simulink model "TestCollecteurAdmissionNew"  (R2025a)
settings: Solver=ode45  StartTime=0.0  StopTime=TempsMaxEvt  MaxStep=0.1  RelTol=1e-9  EnableMultiTasking=on
undefined symbols (not defined in the file): DebitAirEvt, DebitMoteurEvt, ManifoldMassTest, ManifoldPressureTest, ManifoldTemperatureTest, ManifoldTimeTest, Mim0, P0, Tamb, TempsEvt
settings Model: Creator=a030141  LastModifiedBy=Hugo
settings SolverCC: AlgebraicLoopSolver=TrustRegion
settings DataIOCC: LimitDataPoints=on  SaveFormat=Array  SignalLoggingSaveFormat=ModelDataLogs  ReturnWorkspaceOutputs=off  SignalLoggingName=sigsOut
settings OptimizationCC: InitFltsAndDblsToZero=on  LifeSpan=inf
settings DebuggingCC: SaveWithParameterizedLinksMsg=none  UnderspecifiedInitializationDetection=Classic  MergeDetectMultiDrivingBlocksExec=none  SignalResolutionControl=TryResolveAllWithWarning  MultiTaskDSMMsg=warning  MultiTaskCondExecSysMsg=none  FcnCallInpInsideContextMsg=warning  UnconnectedInputMsg=warning  UnconnectedOutputMsg=warning  UnconnectedLineMsg=warning  SFUnexpectedBacktrackingDiag=warning  SFNoUnconditionalDefaultTransitionDiag=warning  SFExecutionAtInitializationDiag=none  ArithmeticOperatorsInVariantConditions=warning
settings HardwareCC: ProdBitPerPointer=32.0  ProdBitPerSizeT=32.0  ProdBitPerPtrDiffT=32.0  ProdLargestAtomicFloat=None  ProdIntDivRoundTo=Undefined  ProdEndianess=Unspecified  ProdWordSize=32.0  ProdHWDeviceType=32-bit Generic  TargetUnknown=on
settings ModelReferenceCC: PropagateSignalLabelsOutOfModel=off
settings RTWCC: GPUComputeCapability=3.5
settings CodeAppCC: StateflowObjectComments=on
settings GRTTargetCC: TargetFcnLib=ansi_tfl_tmw.mat  TargetLangStandard=C89/C90 (ANSI)  CombineOutputUpdateFcns=off  GRTInterface=on
settings ConfigComp: CovMetricSettings=dw  CovSaveCumulativeToWorkspaceVar=on  CovSaveSingleToWorkspaceVar=on

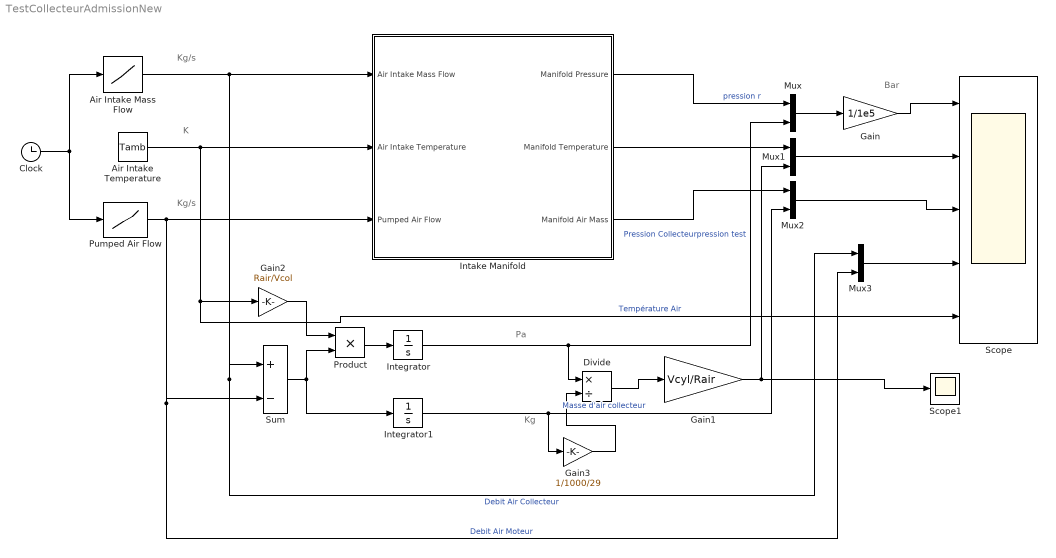
== system TestCollecteurAdmissionNew ==
  note: Kg/s
  note: Kg/s
  note: K
  note: Kg
  note: Pa
  note: Bar
  Air Intake Mass Flow : Lookup  InputValues=TempsEvt  Table=DebitAirEvt
  Air Intake Temperature : Constant  Value=Tamb
  Clock : Clock
  Divide : Product  Inputs=*/
  Gain : Gain  Gain=1/1e5  SaturateOnIntegerOverflow=on  OutDataTypeStr=Inherit: Same as input  ParamDataTypeStr=Inherit: Same as input
  Gain1 : Gain  Gain=Vcyl/Rair
  Gain2 : Gain  Gain=Rair/Vcol
  Gain3 : Gain  Gain=1/1000/29
  Intake Manifold : Subsystem
  Integrator : Integrator  InitialCondition=P0
  Integrator1 : Integrator  InitialCondition=Mim0
  Mux{,1..3} (4 alike) : Mux  Inputs=2
  Product : Product
  Pumped Air Flow : Lookup  InputValues=TempsEvt  Table=DebitMoteurEvt
  Scope : Scope  NumInputPorts=5
      settings: Title=Pression [Bar]  ActiveDisplayYMinimum=-0.308572555020314  ActiveDisplayYMaximum=3.625488784492187
  Scope1 : Scope
      settings: ActiveDisplayYMinimum=1.2162577237181367  ActiveDisplayYMaximum=1.2496676340070305
  Sum : Sum  Inputs=|+-
  wires:
  Integrator/1 -> Divide/1, Mux/2  "Pression Collecteurpression test"
  Clock/1 -> Pumped Air Flow/1, Air Intake Mass Flow/1
  Air Intake Mass Flow/1 -> Mux3/1, Sum/1, Intake Manifold/1(Air Intake Mass Flow)  "Debit Air Collecteur"
  Pumped Air Flow/1 -> Mux3/2, Sum/2, Intake Manifold/3(Pumped Air Flow)  "Debit Air Moteur"
  Air Intake Temperature/1 -> Gain2/1, Scope/5, Intake Manifold/2(Air Intake Temperature)  "Température Air"
  Mux/1 -> Gain/1
  Gain/1 -> Scope/1
  Mux1/1 -> Scope/2
  Mux2/1 -> Scope/3
  Mux3/1 -> Scope/4
  Intake Manifold/1(Manifold Pressure) -> Mux/1  "pression r"
  Intake Manifold/3(Manifold Air Mass) -> Mux2/1
  Product/1 -> Integrator/1
  Sum/1 -> Integrator1/1, Product/2
  Gain2/1 -> Product/1
  Integrator1/1 -> Gain3/1, Mux2/2  "Masse d'air collecteur"
  Intake Manifold/2(Manifold Temperature) -> Mux1/1
  Divide/1 -> Gain1/1
  Gain3/1 -> Divide/2
  Gain1/1 -> Scope1/1, Mux1/2

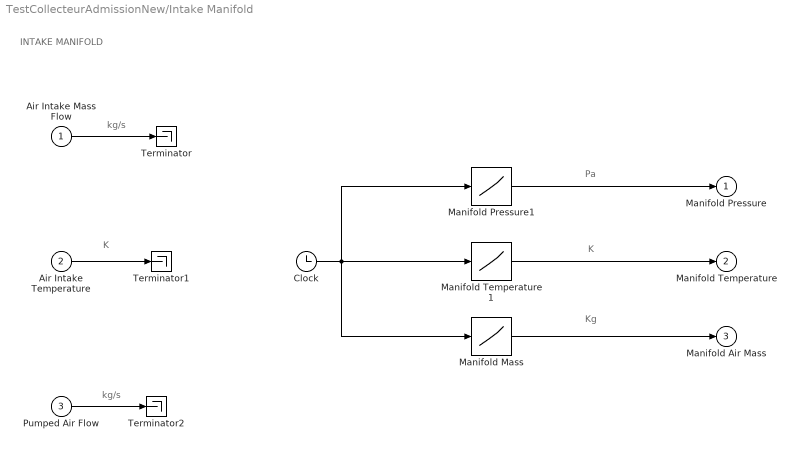
== system TestCollecteurAdmissionNew/Intake Manifold ==
  note: INTAKE MANIFOLD
  note: kg/s
  note: K
  note: kg/s
  note: Kg
  note: K
  note: Pa
  Air Intake Mass Flow : Inport
  Air Intake Temperature : Inport  Port=2
  Pumped Air Flow : Inport  Port=3
  Clock : Clock
  Manifold Mass : Lookup  InputValues=ManifoldTimeTest  Table=ManifoldMassTest
  Manifold Pressure1 : Lookup  InputValues=ManifoldTimeTest  Table=ManifoldPressureTest
  Manifold Temperature1 : Lookup  InputValues=ManifoldTimeTest  Table=ManifoldTemperatureTest
  Terminator : Terminator
  Terminator1 : Terminator
  Terminator2 : Terminator
  Manifold Pressure : Outport
  Manifold Temperature : Outport  Port=2
  Manifold Air Mass : Outport  Port=3
  wires:
  Pumped Air Flow/1 -> Terminator2/1
  Air Intake Mass Flow/1 -> Terminator/1
  Air Intake Temperature/1 -> Terminator1/1
  Manifold Pressure1/1 -> Manifold Pressure/1
  Manifold Temperature1/1 -> Manifold Temperature/1
  Manifold Mass/1 -> Manifold Air Mass/1
  Clock/1 -> Manifold Temperature1/1, Manifold Pressure1/1, Manifold Mass/1
